simulink model "power_converter"  (Simulink 6.0)
settings: Solver=ode23tb  SolverMode=SingleTasking  StartTime=0.0  StopTime=.1  RelTol=1e-3
libraries: powerlib x18, powerlib_extras x1
settings Model: Creator=sybille  LastModifiedBy=batserve  ExtModeTrigMode=oneshot  ExtModeArmWhenConnect=off  ExtModeAutoUpdateStatusClock=off
settings SolverCC: MaxOrder=1
settings DataIOCC: LimitDataPoints=off  SaveOutput=off  SaveTime=off  SignalLoggingName=sigsOut
settings OptimizationCC: BlockReduction=off  BooleanDataType=off
settings DebuggingCC: CheckExecutionContextPreStartOutputMsg=on  CheckExecutionContextRuntimeOutputMsg=on  SolverPrmCheckMsg=none  UnconnectedInputMsg=none  UnconnectedOutputMsg=none
settings HardwareCC: TargetUnknown=on
settings RTWCC: TemplateMakefile=grt_unix.tmf

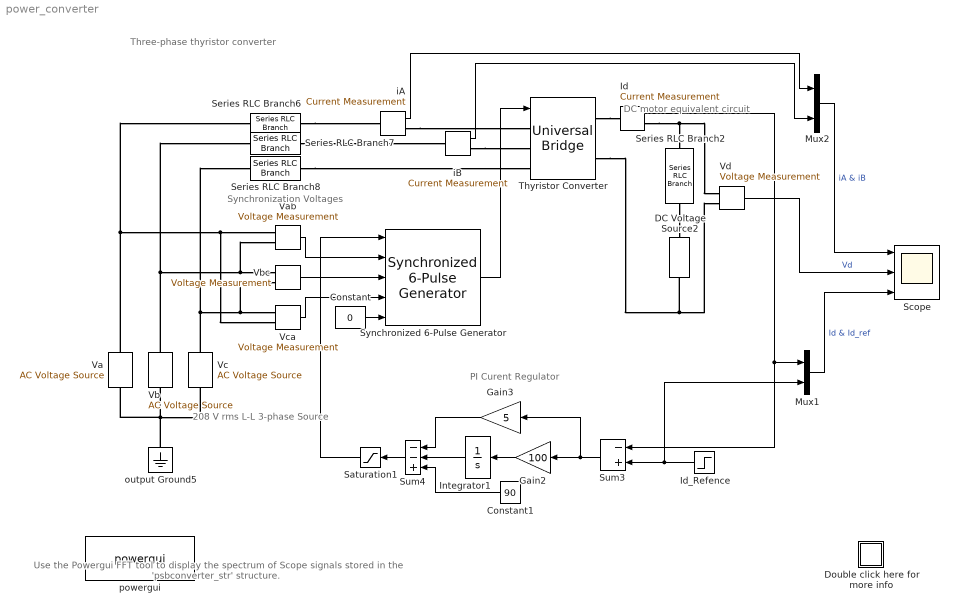
== system power_converter ==
  note: Synchronization Voltages
  note: DC motor equivalent circuit
  note: PI Curent Regulator
  note: Three-phase thyristor converter
  note: 208 V rms L-L
      | 3-phase Source
  note: Use the Powergui FFT tool to display
      | the spectrum of Scope  signals stored in
      | the 'psbconverter_str' structure.
  Constant : Constant  Value=0
  Constant1 : Constant  Orientation=left  Value=90
  DC Voltage Source2 : powerlib/Electrical Sources/DC Voltage Source  Description=source block  Orientation=up  Amplitude=120  Measurements=None
      settings: AttributesFormatString=\n
  Double click here for more info : Subsystem
      mask Display: disp('?')
  Gain2 : Gain  Orientation=left  Gain=100  SaturateOnIntegerOverflow=on
  Gain3 : Gain  Orientation=left  Gain=5  SaturateOnIntegerOverflow=on
  Id : powerlib/Measurements/Current Measurement  Tag=PoWeRsYsTeMmEaSuReMeNt  PhasorSimulation=off  OutputType=Complex  PSBequivalent=0
  Id_Refence : Step  Orientation=left  Time=0.04  Before=10  After=25  SampleTime=0
  Integrator1 : Integrator  Orientation=left  InitialCondition=20  LimitOutput=on  UpperSaturationLimit=160  LowerSaturationLimit=20
  Mux1 : Mux  Inputs=2
  Mux2 : Mux  Inputs=2
  Saturation1 : Saturate  Orientation=left  UpperLimit=160  LowerLimit=20
  Scope : Scope  NumInputPorts=3
      settings: TimeRange=0.1  YMin=-50~-200~-3.20216e-017  YMax=50~400~40  SaveName=psbconverter_str  SampleInput=on  SampleTime=1/60/512
  Series RLC Branch2 : powerlib/Elements/Series RLC Branch  Orientation=down  PhysicalDomain=powersysdomain  SubClassName=unknown  LeftPortType=p1  RightPortType=p1  LConnTagsString=__new0  RConnTagsString=__new0  Resistance=1  Inductance=20e-3  Capacitance=inf  Measurements=None
  Series RLC Branch6 : powerlib/Elements/Series RLC Branch  PhysicalDomain=powersysdomain  SubClassName=unknown  LeftPortType=p1  RightPortType=p1  LConnTagsString=__new0  RConnTagsString=__new0  Resistance=0.01  Inductance=1e-3  Capacitance=inf  Measurements=None
  Series RLC Branch7 : powerlib/Elements/Series RLC Branch  PhysicalDomain=powersysdomain  SubClassName=unknown  LeftPortType=p1  RightPortType=p1  LConnTagsString=__new0  RConnTagsString=__new0  Resistance=0.01  Inductance=1e-3  Capacitance=inf  Measurements=None
  Series RLC Branch8 : powerlib/Elements/Series RLC Branch  PhysicalDomain=powersysdomain  SubClassName=unknown  LeftPortType=p1  RightPortType=p1  LConnTagsString=__new0  RConnTagsString=__new0  Resistance=0.01  Inductance=1e-3  Capacitance=inf  Measurements=None
  Sum3 : Sum  Orientation=left  Inputs=-+  SaturateOnIntegerOverflow=on  InputSameDT=on
  Sum4 : Sum  Orientation=left  Inputs=--+  SaturateOnIntegerOverflow=on  InputSameDT=on
  Synchronized 6-Pulse Generator : powerlib_extras/Control  Blocks/Synchronized 6-Pulse Generator  freq=60  pwidth=10  Double_Pulse=on
  Thyristor Converter : powerlib/Power Electronics/Universal Bridge  Arms=3  SnubberResistance=500  SnubberCapacitance=.1e-6  Device=Thyristors  Ron=1e-3  Lon=0  ForwardVoltages="[  0.8  0.8  ]"  ForwardVoltage=.8  GTOparameters=[ 10e-6 , 20e-6 ]  IGBTparameters=[ 1e-6 , 2e-6 ]  Measurements=None
  Va : powerlib/Electrical Sources/AC Voltage Source  Description=source block  Orientation=up  Amplitude=208*sqrt(2/3)  Phase=0  Frequency=60  SampleTime=0  Measurements=None
      settings: AttributesFormatString=\n
  Vab : powerlib/Measurements/Voltage Measurement  Tag=PoWeRsYsTeMmEaSuReMeNt  PhasorSimulation=off  OutputType=Complex  PSBequivalent=0
  Vb : powerlib/Electrical Sources/AC Voltage Source  Description=source block  Orientation=up  Amplitude=208*sqrt(2/3)  Phase=-120  Frequency=60  SampleTime=0  Measurements=None
      settings: AttributesFormatString=\n
  Vbc : powerlib/Measurements/Voltage Measurement  Tag=PoWeRsYsTeMmEaSuReMeNt  PhasorSimulation=off  OutputType=Complex  PSBequivalent=0
  Vc : powerlib/Electrical Sources/AC Voltage Source  Description=source block  Orientation=up  Amplitude=208*sqrt(2/3)  Phase=120  Frequency=60  SampleTime=0  Measurements=None
      settings: AttributesFormatString=\n
  Vca : powerlib/Measurements/Voltage Measurement  Tag=PoWeRsYsTeMmEaSuReMeNt  PhasorSimulation=off  OutputType=Complex  PSBequivalent=0
  Vd : powerlib/Measurements/Voltage Measurement  Tag=PoWeRsYsTeMmEaSuReMeNt  PhasorSimulation=off  OutputType=Complex  PSBequivalent=0
  iA : powerlib/Measurements/Current Measurement  Tag=PoWeRsYsTeMmEaSuReMeNt  PhasorSimulation=off  OutputType=Complex  PSBequivalent=0
  iB : powerlib/Measurements/Current Measurement  Tag=PoWeRsYsTeMmEaSuReMeNt  PhasorSimulation=off  OutputType=Complex  PSBequivalent=0
  output Ground5 : powerlib/Elements/Ground  Orientation=down  PhysicalDomain=powersysdomain  SubClassName=unknown  LeftPortType=p1  RightPortType=p1  LConnTagsString=a
  powergui : powerlib/powergui  Priority=2  Frange=[0:2:500]  Ylog=off  Xlog=on  save=off  variable=ZData  structure=psbconverter_str  ZoomFFT=on  StartTime=0.1-2/60  cycles=2  DisplayStyle=off  fundamental=60  FreqAxis=on  MaxFrequency=2000  frequencyindice=1  frequencyindicesteady=1  RmsSteady=1  display=off  Ts=0  methode=off  frequency=60  echomessages=on
  wires:
  Gain3/1 -> Sum4/1
  Constant1/1 -> Sum4/3
  Gain2/1 -> Integrator1/1
  Sum3/1 -> Gain3/1, Gain2/1
  Sum4/1 -> Saturation1/1
  Integrator1/1 -> Sum4/2
  Saturation1/1 -> Synchronized 6-Pulse Generator/1
  Id_Refence/1 -> Sum3/2, Mux1/2
  Mux2/1 -> Scope/1  "iA & iB"
  Mux1/1 -> Scope/3  "Id & Id_ref"
  Constant/1 -> Synchronized 6-Pulse Generator/5
  Id/1 -> Mux1/1, Sum3/1
  Vca/1 -> Synchronized 6-Pulse Generator/4
  Vbc/1 -> Synchronized 6-Pulse Generator/3
  Vab/1 -> Synchronized 6-Pulse Generator/2
  iA/1 -> Mux2/1
  iB/1 -> Mux2/2
  Vd/1 -> Scope/2  "Vd"
  Synchronized 6-Pulse Generator/1 -> Thyristor Converter/1
  connections:
  Thyristor Converter/RConn1 -- Id/LConn1
  output Ground5/LConn1 -- Vb/LConn1 -- Va/LConn1 -- Vc/LConn1
  Id/RConn1 -- Series RLC Branch2/LConn1 -- Vd/LConn1
  Series RLC Branch2/RConn1 -- DC Voltage Source2/RConn1
  Vb/RConn1 -- Vbc/LConn1 -- Vab/LConn2 -- Series RLC Branch7/LConn1
  Vc/RConn1 -- Vca/LConn1 -- Vbc/LConn2 -- Series RLC Branch8/LConn1
  Va/RConn1 -- Vab/LConn1 -- Vca/LConn2 -- Series RLC Branch6/LConn1
  Series RLC Branch8/RConn1 -- Thyristor Converter/LConn3
  Series RLC Branch6/RConn1 -- iA/LConn1
  iA/RConn1 -- Thyristor Converter/LConn1
  Series RLC Branch7/RConn1 -- iB/LConn1
  iB/RConn1 -- Thyristor Converter/LConn2
  Thyristor Converter/RConn2 -- DC Voltage Source2/LConn1 -- Vd/LConn2

== system power_converter/Double click here for more info ==
  note: This demonstration illustrates use of the Universal Bridge block to simulate a three-phase six-pulse
      | converter and harmonic analysis using the Powergui/FFT tool.
  note: Circuit Description
  note: A  DC motor  represented by a simplified RL-E model is fed from  an inductive three-phase source through a six-pulse
      | thyristor bridge. A pulse generator synchronized on the source voltages provides the trigger pulses for the six thyristors.
      |
      | The converter output current is controlled by a PI current regulator built with Simulink blocks.
      | A step signal is applied to the reference input to test the dynamic response of the current regulator.
      |
      | In order to allow further signal processing, signals displayed on the Scope block are sampled at 1/60/512 s (512 samples/ cycle) and stored
      | in a variable named 'psbconveter_str'  ('structure with time'  format) .
  note: H. Le-Huy (Universite Laval, Quebec)
  note: Demonstration
  note: Start simulation and observe current and voltage waveforms on the Scope block.
      |
      | When  simulation is completed, open the Powergui and select  'FFT Analysis' to display the 0 - 2000 Hz frequency spectrum of signals saved
      | in the 'psbconverter_str' structure. The FFT will be performed on  a 2-cycle window starting at t = 0.1 - 2/60 (last 2 cycles of recording).
      | Input labeled 'Ia & Ib' and signal number 1 (Ia) should be already selected. Click on Display and observe the frequency spectrum of last two cycles of Ia.
      | Harmonic currents (6n+/-1) are displayed in % of the fundamental component .
      |
      | The value of the fundamental current (magnitude = 27.48 A peak) and the Total Harmonic Distortion (THD) are also displayed.
      | Harrmonics in the 0 - 2000 Hz range contribute to 29% in THD. If you specify a 0-4000 Hz frequence range, notice that
      | contributions of harmonics above 2000 Hz are negligible in the current THD.
      |
      | Now select the input labeled Vd and display its spectrum.
      | The DC voltage contains harmonics (6n) and its DC component is 145.4 V.
